simulink model "ElectricalThermalSystemSSC"  (R2026b)
settings: Solver=VariableStepAuto
undefined symbols (not defined in the file): coolant_pipe_D, coolant_valve_D_ratio_max, coolant_valve_D_ratio_min, coolant_valve_displacement, EnvAirTemp, EnvGrvty, PlntThrCabCO2Init, PlntThrCabDucArea, PlntThrCabFanMaxFlw, PlntThrCabHtc, PlntThrCabNPass, PlntThrCabRelHInit, PlntThrCabTempAvg, PlntThrChArea, PlntThrCmpMaxSpd, PlntThrCoolTnkArea, PlntThrCoolTnkVol, PlntThrDoorsArea, PlntThrDoorsK, PlntThrDoorsTk, PlntThrExpDia, PlntThrFanMaxSpd, PlntThrFanMechEff, PlntThrFanVolEff, PlntThrGlassArea, PlntThrGlassK, PlntThrGlassTk, PlntThrHeaterMaxPwr, PlntThrHexNTubes, PlntThrHexTubeDia, PlntThrPipeArea, PlntThrPipeDia, PlntThrPmpMaxSpd, PlntThrPTCLimTemp, PlntThrPTCPwrGain, PlntThrRefrigDia, PlntThrRefrigPinit, PlntThrRoofArea, PlntThrRoofK, PlntThrRoofTk, PlntThrValDisp, PlntThrValDratioMax, PlntThrValDratioMin, PlntThrValRefrDisp, PlntThrValRefrDratio, PlntThrValSplMax, ThrmEM1, ThrmEM2, ThrmEM3, ThrmEM4
libraries: fl_lib x149, nesl_utility x81, SimscapeFluids_lib x35, autolibutils x21
(part 1 of 6)
settings Model: ModifiedByFormat=The MathWorks, Inc.  Creator=The MathWorks, Inc.  LastModifiedBy=The MathWorks, Inc.

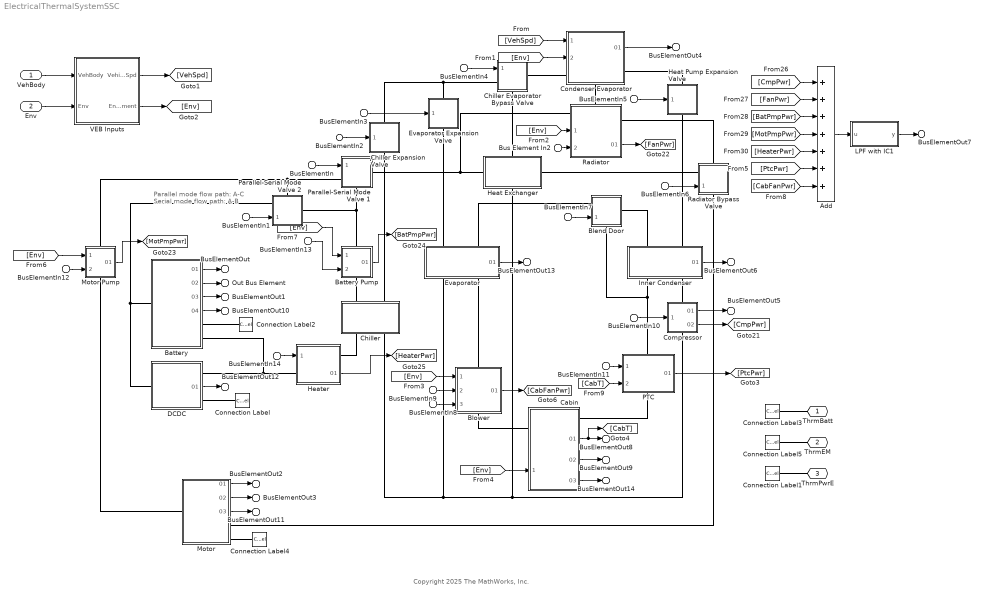
== system ElectricalThermalSystemSSC ==
  note: Parallel mode flow path: A-C
      | Serial mode flow path: A-B
  note: Copyright 2025 The MathWorks, Inc.
  VehBody : Inport
  Env : Inport  Port=2
  BusElementIn10 : Inport  Port=3  PortName=Cntrl  Element=Thermal.CmpCmd
  Bus Element In2 : Inport  Port=3  PortName=Cntrl  Element=Thermal.FanCmd
  BusElementIn14 : Inport  Port=3  PortName=Cntrl  Element=Thermal.HeaterCmd
  BusElementIn12 : Inport  Port=3  PortName=Cntrl  Element=Thermal.MotPmpCmd
  BusElementIn13 : Inport  Port=3  PortName=Cntrl  Element=Thermal.BattPmpCmd
  BusElementIn : Inport  Port=3  PortName=Cntrl  Element=Thermal.SerParCmd
  BusElementIn1 : Inport  Port=3  PortName=Cntrl  Element=Thermal.SerParCmd
  BusElementIn6 : Inport  Port=3  PortName=Cntrl  Element=Thermal.RadByPCmd
  BusElementIn9 : Inport  Port=3  PortName=Cntrl  Element=Thermal.CabFanCmd
  BusElementIn8 : Inport  Port=3  PortName=Cntrl  Element=Thermal.RecircCmd
  BusElementIn11 : Inport  Port=3  PortName=Cntrl  Element=Thermal.PtcCmd
  BusElementIn4 : Inport  Port=3  PortName=Cntrl  Element=Thermal.RfrgByPCmd
  BusElementIn7 : Inport  Port=3  PortName=Cntrl  Element=Thermal.BlndAirCmd
  BusElementIn2 : Inport  Port=3  PortName=Cntrl  Element=Thermal.ChlrXCmd
  BusElementIn3 : Inport  Port=3  PortName=Cntrl  Element=Thermal.AcCmd
  BusElementIn5 : Inport  Port=3  PortName=Cntrl  Element=Thermal.HpXCmd
  Add : Sum  Inputs=+++++++
  Battery : Subsystem  Tag=PublishSubsystem  VariantControl=Mapped
      mask Display: disp(get_param(gcb, 'Name'))
  Battery Pump : Subsystem
      settings: PortSchema="{\"entries\":[{\"content\":{\"sides\":[{\"content\":{\"connectorIds\":[\"In1\",\"In2\"]},\"type\":\"ConnectorPlacement.EquallySpacedRectSide\",\"uuid\":\"8608e54e-2c97-4e6c-91d5-e9fd83f4c634\"},{\"content\":{\"connectorIds\":[\"Out1\"],\"side\":\"RIGHT\"},\"type\":\"ConnectorPlacement.EquallySpacedRectSide\",\"uuid\":\"2094794e-7928-4a36-8d26-6d0877832239\"},{\"content\":{\"connectorIds\":[\"LConn1\"],\"side\":\"TOP\"},\"type\":\"ConnectorPlacement.EquallySpacedRectSide\",\"uuid\":\"5d2e6c3a-6919-4acd-9f23-628827b4d5b1\"},{\"content\":{\"connectorIds\":[\"RConn1\"],\"side\":\"BOTTOM\"},\"type\":\"ConnectorPlacement.EquallySpacedRectSide\",\"uuid\":\"7eb8f1d1-21e2-47d8-bcb5-892664c8f83c\"}]},\"type\":\"ConnectorPlacement.EquallySpacedConnector\",\"uuid\":\"45db803b-5189-4980-a07c-fba0b10a9ca2\"}],\"packageUris\":[\"http://schema.mathworks.com/mf0/Connector/R2020b\"],\"version\":\"1.0\"}"
      mask Display:
      | plot(100*cos(linspace(0, 2*pi, 500)), 100*sin(linspace(0, 2*pi, 500)))
      | patch([0 24 -24 0], [-100 -55 -55 -100]+1, [0 0 0])
  Blend Door : Subsystem
      settings: PortSchema="{\"entries\":[{\"content\":{\"sides\":[{\"content\":{\"connectorIds\":[\"LConn1\",\"In1\"]},\"type\":\"ConnectorPlacement.EquallySpacedRectSide\",\"uuid\":\"8608e54e-2c97-4e6c-91d5-e9fd83f4c634\"},{\"content\":{\"connectorIds\":[\"RConn1\"],\"side\":\"RIGHT\"},\"type\":\"ConnectorPlacement.EquallySpacedRectSide\",\"uuid\":\"2094794e-7928-4a36-8d26-6d0877832239\"},{\"content\":{\"side\":\"TOP\"},\"type\":\"ConnectorPlacement.EquallySpacedRectSide\",\"uuid\":\"5d2e6c3a-6919-4acd-9f23-628827b4d5b1\"},{\"content\":{\"connectorIds\":[\"RConn2\"],\"side\":\"BOTTOM\"},\"type\":\"ConnectorPlacement.EquallySpacedRectSide\",\"uuid\":\"12f1c895-2983-4276-b305-f1b4f2b8f289\"}]},\"type\":\"ConnectorPlacement.EquallySpacedConnector\",\"uuid\":\"45db803b-5189-4980-a07c-fba0b10a9ca2\"}],\"packageUris\":[\"http://schema.mathworks.com/mf0/Connector/R2020b\"],\"version\":\"1.0\"}"
      mask Display:
      | color('white')
      | plot(100, 100)
      | plot(-100, -100)
      | color('black')
      | 
      | plot([0 -100 -100 0], [0 50 -50 0])
      | plot([0 100 100 0], [0 50 -50 0])
      | plot([0 50 -50 0], [0 -100 -100 0])
  Blower : Subsystem  Tag=PublishSubsystem
      settings: PortSchema="{\"entries\":[{\"content\":{\"sides\":[{\"content\":{\"connectorIds\":[\"In1\",\"In2\",\"In3\"]},\"type\":\"ConnectorPlacement.EquallySpacedRectSide\",\"uuid\":\"9f1db8dd-3953-4c85-b0fd-c908a14d75c2\"},{\"content\":{\"connectorIds\":[\"Out1\"],\"side\":\"RIGHT\"},\"type\":\"ConnectorPlacement.EquallySpacedRectSide\",\"uuid\":\"6831d28e-85a7-47d3-a33b-c75afeea3e4b\"},{\"content\":{\"connectorIds\":[\"LConn1\"],\"side\":\"TOP\"},\"type\":\"ConnectorPlacement.EquallySpacedRectSide\",\"uuid\":\"f6a34470-b429-4b8f-bc43-b876cd933588\"},{\"content\":{\"connectorIds\":[\"RConn1\"],\"side\":\"BOTTOM\"},\"type\":\"ConnectorPlacement.EquallySpacedRectSide\",\"uuid\":\"65552e63-bdf8-40c1-9881-c42b86485e87\"}]},\"type\":\"ConnectorPlacement.EquallySpacedConnector\",\"uuid\":\"95b80f6b-f2a0-41c8-b218-6929a9df8903\"}],\"packageUris\":[\"http://schema.mathworks.com/mf0/Connector/R2020b\"],\"version\":\"1.0\"}"
      mask Display:
      | plot(100*cos(linspace(0, 2*pi, 500)), 100*sin(linspace(0, 2*pi, 500)))
      | plot([28 80], [96 -60])
      | plot([-28 -80], [96 -60])
      | patch(-50*sin(3*linspace(0, pi, 500)).*cos(linspace(0, pi, 500)), -50*sin(3*linspace(0, pi, 500)).*sin(linspace(0, pi, 500)), [0 0 0])
  Cabin : Subsystem  Tag=PublishSubsystem
      settings: PortSchema="{\"entries\":[{\"content\":{\"sides\":[{\"content\":{\"connectorIds\":[\"LConn1\",\"In1\"]},\"type\":\"ConnectorPlacement.EquallySpacedRectSide\",\"uuid\":\"20781a4d-44d2-4d8b-9b82-72093275c353\"},{\"content\":{\"connectorIds\":[\"RConn1\",\"Out1\",\"Out2\",\"Out3\"],\"side\":\"RIGHT\"},\"type\":\"ConnectorPlacement.EquallySpacedRectSide\",\"uuid\":\"764c44ca-e93e-4bde-bd39-740c4b6195f1\"},{\"content\":{\"side\":\"TOP\"},\"type\":\"ConnectorPlacement.EquallySpacedRectSide\",\"uuid\":\"542c8f7d-7f76-4cb4-898c-a40529f31b50\"}]},\"type\":\"ConnectorPlacement.EquallySpacedConnector\",\"uuid\":\"d0ad0532-a708-440a-8350-71ab63903cc5\"}],\"packageUris\":[\"http://schema.mathworks.com/mf0/Connector/R2020b\"],\"version\":\"1.0\"}"
      mask Display: disp(get_param(gcb, 'Name'))
  Chiller : Subsystem  Tag=PublishSubsystem
      settings: PortSchema="{\"entries\":[{\"content\":{\"sides\":[{\"content\":{},\"type\":\"ConnectorPlacement.EquallySpacedRectSide\",\"uuid\":\"08dd7f1a-2c57-4e0b-bc0c-3dc595a62f47\"},{\"content\":{\"side\":\"RIGHT\"},\"type\":\"ConnectorPlacement.EquallySpacedRectSide\",\"uuid\":\"ff3adbe6-50e6-4ee9-89c8-33b172e39e14\"},{\"content\":{\"connectorIds\":[\"LConn1\",\"LConn2\"],\"side\":\"TOP\"},\"type\":\"ConnectorPlacement.EquallySpacedRectSide\",\"uuid\":\"dbd0f117-c61e-4d8b-a34c-15c789eeb10d\"},{\"content\":{\"connectorIds\":[\"RConn1\",\"RConn2\"],\"side\":\"BOTTOM\"},\"type\":\"ConnectorPlacement.EquallySpacedRectSide\",\"uuid\":\"0d4c84fc-b13c-4ee0-9956-2ee11d67b2ad\"}]},\"type\":\"ConnectorPlacement.EquallySpacedConnector\",\"uuid\":\"74c2ffb8-8fce-48fb-ac7c-d547444760e2\"}],\"packageUris\":[\"http://schema.mathworks.com/mf0/Connector/R2020b\"],\"version\":\"1.0\"}"
      mask Display: disp(get_param(gcb, 'Name'))
  Chiller Expansion Valve : Subsystem  Tag=PublishSubsystem
      settings: PortSchema="{\"entries\":[{\"content\":{\"sides\":[{\"content\":{\"connectorIds\":[\"In1\"]},\"type\":\"ConnectorPlacement.EquallySpacedRectSide\",\"uuid\":\"8608e54e-2c97-4e6c-91d5-e9fd83f4c634\"},{\"content\":{\"side\":\"RIGHT\"},\"type\":\"ConnectorPlacement.EquallySpacedRectSide\",\"uuid\":\"2094794e-7928-4a36-8d26-6d0877832239\"},{\"content\":{\"connectorIds\":[\"LConn1\"],\"side\":\"TOP\"},\"type\":\"ConnectorPlacement.EquallySpacedRectSide\",\"uuid\":\"5d2e6c3a-6919-4acd-9f23-628827b4d5b1\"},{\"content\":{\"connectorIds\":[\"RConn1\"],\"side\":\"BOTTOM\"},\"type\":\"ConnectorPlacement.EquallySpacedRectSide\",\"uuid\":\"5466525f-0f04-4dbe-888f-4c3dddfbc528\"}]},\"type\":\"ConnectorPlacement.EquallySpacedConnector\",\"uuid\":\"45db803b-5189-4980-a07c-fba0b10a9ca2\"}],\"packageUris\":[\"http://schema.mathworks.com/mf0/Connector/R2020b\"],\"version\":\"1.0\"}"
      mask Display:
      | color('white')
      | plot(100, 100)
      | plot(-100, -100)
      | color('black')
      | 
      | plot([0 50 -50 0], [0 -100 -100 0])
      | plot([0 50 -50 0], [0 100 100 0])
  Chiller Evaporator Bypass Valve : Subsystem  Tag=PublishSubsystem
      settings: PortSchema="{\"entries\":[{\"content\":{\"sides\":[{\"content\":{\"connectorIds\":[\"In1\",\"LConn1\"]},\"type\":\"ConnectorPlacement.EquallySpacedRectSide\",\"uuid\":\"8608e54e-2c97-4e6c-91d5-e9fd83f4c634\"},{\"content\":{\"connectorIds\":[\"RConn1\"],\"side\":\"RIGHT\"},\"type\":\"ConnectorPlacement.EquallySpacedRectSide\",\"uuid\":\"2094794e-7928-4a36-8d26-6d0877832239\"},{\"content\":{\"side\":\"TOP\"},\"type\":\"ConnectorPlacement.EquallySpacedRectSide\",\"uuid\":\"5d2e6c3a-6919-4acd-9f23-628827b4d5b1\"},{\"content\":{\"connectorIds\":[\"RConn2\"],\"side\":\"BOTTOM\"},\"type\":\"ConnectorPlacement.EquallySpacedRectSide\",\"uuid\":\"12f1c895-2983-4276-b305-f1b4f2b8f289\"}]},\"type\":\"ConnectorPlacement.EquallySpacedConnector\",\"uuid\":\"45db803b-5189-4980-a07c-fba0b10a9ca2\"}],\"packageUris\":[\"http://schema.mathworks.com/mf0/Connector/R2020b\"],\"version\":\"1.0\"}"
      mask Display:
      | color('white')
      | plot(100, 100)
      | plot(-100, -100)
      | color('black')
      | 
      | plot([0 -100 -100 0], [0 50 -50 0])
      | plot([0 100 100 0], [0 50 -50 0])
      | plot([0 50 -50 0], [0 -100 -100 0])
  Compressor : Subsystem  Tag=PublishSubsystem
      settings: PortSchema="{\"entries\":[{\"content\":{\"sides\":[{\"content\":{\"connectorIds\":[\"In1\"]},\"type\":\"ConnectorPlacement.EquallySpacedRectSide\",\"uuid\":\"8608e54e-2c97-4e6c-91d5-e9fd83f4c634\"},{\"content\":{\"connectorIds\":[\"Out1\",\"Out2\"],\"side\":\"RIGHT\"},\"type\":\"ConnectorPlacement.EquallySpacedRectSide\",\"uuid\":\"2094794e-7928-4a36-8d26-6d0877832239\"},{\"content\":{\"connectorIds\":[\"LConn1\"],\"side\":\"TOP\"},\"type\":\"ConnectorPlacement.EquallySpacedRectSide\",\"uuid\":\"5d2e6c3a-6919-4acd-9f23-628827b4d5b1\"},{\"content\":{\"connectorIds\":[\"RConn1\"],\"side\":\"BOTTOM\"},\"type\":\"ConnectorPlacement.EquallySpacedRectSide\",\"uuid\":\"ed0a8ac6-4625-4be3-8c8e-84380e16051c\"}]},\"type\":\"ConnectorPlacement.EquallySpacedConnector\",\"uuid\":\"45db803b-5189-4980-a07c-fba0b10a9ca2\"}],\"packageUris\":[\"http://schema.mathworks.com/mf0/Connector/R2020b\"],\"version\":\"1.0\"}"
      mask Display:
      | plot(100*cos(linspace(0, 2*pi, 500)), 100*sin(linspace(0, 2*pi, 500)))
      | plot([28 80], [96 -60])
      | plot([-28 -80], [96 -60])
  Condenser Evaporator : Subsystem  Tag=PublishSubsystem
      settings: PortSchema="{\"entries\":[{\"content\":{\"sides\":[{\"content\":{\"connectorIds\":[\"In1\",\"In2\",\"LConn1\"]},\"type\":\"ConnectorPlacement.EquallySpacedRectSide\",\"uuid\":\"07c3df60-ca73-4a82-8a74-bbe62fbe14d4\"},{\"content\":{\"connectorIds\":[\"Out1\",\"RConn1\"],\"side\":\"RIGHT\"},\"type\":\"ConnectorPlacement.EquallySpacedRectSide\",\"uuid\":\"9db9ae49-9d94-4ce4-9f2f-75754f4c26b5\"},{\"content\":{\"side\":\"TOP\"},\"type\":\"ConnectorPlacement.EquallySpacedRectSide\",\"uuid\":\"fd8c0c23-133d-46ca-bac8-f53d714a10c9\"},{\"content\":{\"connectorIds\":[\"RConn2\"],\"side\":\"BOTTOM\"},\"type\":\"ConnectorPlacement.EquallySpacedRectSide\",\"uuid\":\"1982af02-f04e-4e44-9cd8-4410768eed4d\"}]},\"type\":\"ConnectorPlacement.EquallySpacedConnector\",\"uuid\":\"8e0ae7db-f1f8-46e5-b300-69983ccb91b0\"}],\"packageUris\":[\"http://schema.mathworks.com/mf0/Connector/R2020b\"],\"version\":\"1.0\"}"
      mask Display: disp(get_param(gcb, 'Name'))
  Connection Label : ConnectionLabel  Label=ThrmPwrE
  Connection Label1 : ConnectionLabel  Label=ThrmPwrE
  Connection Label2 : ConnectionLabel  Label=ThrmBatt
  Connection Label3 : ConnectionLabel  Label=ThrmBatt
  Connection Label4 : ConnectionLabel  Label=ThrmEM
  Connection Label5 : ConnectionLabel  Label=ThrmEM
  DCDC : Subsystem
      settings: PortSchema="{\"entries\":[{\"content\":{\"sides\":[{\"content\":{\"connectorIds\":[\"LConn1\"]},\"type\":\"ConnectorPlacement.EquallySpacedRectSide\",\"uuid\":\"39ab4129-79f9-4d3d-8bc5-1c8c0a2ebbde\"},{\"content\":{\"connectorIds\":[\"RConn1\",\"Out1\",\"RConn2\"],\"side\":\"RIGHT\"},\"type\":\"ConnectorPlacement.EquallySpacedRectSide\",\"uuid\":\"b43cfbcd-b0a5-4cd8-a54f-30d93fd1b128\"},{\"content\":{\"side\":\"TOP\"},\"type\":\"ConnectorPlacement.EquallySpacedRectSide\",\"uuid\":\"91742ef5-5184-4832-8e69-68c8acd6160b\"}]},\"type\":\"ConnectorPlacement.EquallySpacedConnector\",\"uuid\":\"413d9595-534c-4f8c-8212-717ae374098d\"}],\"packageUris\":[\"http://schema.mathworks.com/mf0/Connector/R2020b\"],\"version\":\"1.0\"}"
      mask Display: disp(get_param(gcb, 'Name'))
  Evaporator : Subsystem  Tag=PublishSubsystem
      settings: PortSchema="{\"entries\":[{\"content\":{\"sides\":[{\"content\":{},\"type\":\"ConnectorPlacement.EquallySpacedRectSide\",\"uuid\":\"08dd7f1a-2c57-4e0b-bc0c-3dc595a62f47\"},{\"content\":{\"connectorIds\":[\"Out1\"],\"side\":\"RIGHT\"},\"type\":\"ConnectorPlacement.EquallySpacedRectSide\",\"uuid\":\"ff3adbe6-50e6-4ee9-89c8-33b172e39e14\"},{\"content\":{\"connectorIds\":[\"LConn1\",\"LConn2\"],\"side\":\"TOP\"},\"type\":\"ConnectorPlacement.EquallySpacedRectSide\",\"uuid\":\"dbd0f117-c61e-4d8b-a34c-15c789eeb10d\"},{\"content\":{\"connectorIds\":[\"RConn1\",\"RConn2\"],\"side\":\"BOTTOM\"},\"type\":\"ConnectorPlacement.EquallySpacedRectSide\",\"uuid\":\"a1739911-191b-44a6-b898-cc4889767178\"}]},\"type\":\"ConnectorPlacement.EquallySpacedConnector\",\"uuid\":\"74c2ffb8-8fce-48fb-ac7c-d547444760e2\"}],\"packageUris\":[\"http://schema.mathworks.com/mf0/Connector/R2020b\"],\"version\":\"1.0\"}"
      mask Display: disp(get_param(gcb, 'Name'))
  Evaporator Expansion Valve : Subsystem  Tag=PublishSubsystem
      settings: PortSchema="{\"entries\":[{\"content\":{\"sides\":[{\"content\":{\"connectorIds\":[\"In1\"]},\"type\":\"ConnectorPlacement.EquallySpacedRectSide\",\"uuid\":\"8608e54e-2c97-4e6c-91d5-e9fd83f4c634\"},{\"content\":{\"side\":\"RIGHT\"},\"type\":\"ConnectorPlacement.EquallySpacedRectSide\",\"uuid\":\"2094794e-7928-4a36-8d26-6d0877832239\"},{\"content\":{\"connectorIds\":[\"LConn1\"],\"side\":\"TOP\"},\"type\":\"ConnectorPlacement.EquallySpacedRectSide\",\"uuid\":\"5d2e6c3a-6919-4acd-9f23-628827b4d5b1\"},{\"content\":{\"connectorIds\":[\"RConn1\"],\"side\":\"BOTTOM\"},\"type\":\"ConnectorPlacement.EquallySpacedRectSide\",\"uuid\":\"dee56540-0438-4e4d-b3ab-37064a293584\"}]},\"type\":\"ConnectorPlacement.EquallySpacedConnector\",\"uuid\":\"45db803b-5189-4980-a07c-fba0b10a9ca2\"}],\"packageUris\":[\"http://schema.mathworks.com/mf0/Connector/R2020b\"],\"version\":\"1.0\"}"
      mask Display:
      | color('white')
      | plot(100, 100)
      | plot(-100, -100)
      | color('black')
      | 
      | plot([0 50 -50 0], [0 -100 -100 0])
      | plot([0 50 -50 0], [0 100 100 0])
  Heat Exchanger : Subsystem  Tag=PublishSubsystem
      settings: PortSchema="{\"entries\":[{\"content\":{\"sides\":[{\"content\":{\"connectorIds\":[\"LConn1\"]},\"type\":\"ConnectorPlacement.EquallySpacedRectSide\",\"uuid\":\"08dd7f1a-2c57-4e0b-bc0c-3dc595a62f47\"},{\"content\":{\"connectorIds\":[\"RConn1\"],\"side\":\"RIGHT\"},\"type\":\"ConnectorPlacement.EquallySpacedRectSide\",\"uuid\":\"ff3adbe6-50e6-4ee9-89c8-33b172e39e14\"},{\"content\":{\"connectorIds\":[\"LConn2\"],\"side\":\"TOP\"},\"type\":\"ConnectorPlacement.EquallySpacedRectSide\",\"uuid\":\"dbd0f117-c61e-4d8b-a34c-15c789eeb10d\"},{\"content\":{\"connectorIds\":[\"RConn2\"],\"side\":\"BOTTOM\"},\"type\":\"ConnectorPlacement.EquallySpacedRectSide\",\"uuid\":\"042be640-9063-45a3-8f14-0e35b2f9701a\"}]},\"type\":\"ConnectorPlacement.EquallySpacedConnector\",\"uuid\":\"74c2ffb8-8fce-48fb-ac7c-d547444760e2\"}],\"packageUris\":[\"http://schema.mathworks.com/mf0/Connector/R2020b\"],\"version\":\"1.0\"}"
      mask Display: disp(get_param(gcb, 'Name'))
  Heat Pump Expansion Valve : Subsystem  Tag=PublishSubsystem
      settings: PortSchema="{\"entries\":[{\"content\":{\"sides\":[{\"content\":{\"connectorIds\":[\"In1\"]},\"type\":\"ConnectorPlacement.EquallySpacedRectSide\",\"uuid\":\"8608e54e-2c97-4e6c-91d5-e9fd83f4c634\"},{\"content\":{\"side\":\"RIGHT\"},\"type\":\"ConnectorPlacement.EquallySpacedRectSide\",\"uuid\":\"2094794e-7928-4a36-8d26-6d0877832239\"},{\"content\":{\"connectorIds\":[\"LConn1\"],\"side\":\"TOP\"},\"type\":\"ConnectorPlacement.EquallySpacedRectSide\",\"uuid\":\"5d2e6c3a-6919-4acd-9f23-628827b4d5b1\"},{\"content\":{\"connectorIds\":[\"RConn1\"],\"side\":\"BOTTOM\"},\"type\":\"ConnectorPlacement.EquallySpacedRectSide\",\"uuid\":\"a6d8b143-f5c4-47d8-b413-b9e61d8ce1dd\"}]},\"type\":\"ConnectorPlacement.EquallySpacedConnector\",\"uuid\":\"45db803b-5189-4980-a07c-fba0b10a9ca2\"}],\"packageUris\":[\"http://schema.mathworks.com/mf0/Connector/R2020b\"],\"version\":\"1.0\"}"
      mask Display:
      | color('white')
      | plot(100, 100)
      | plot(-100, -100)
      | color('black')
      | 
      | plot([0 50 -50 0], [0 -100 -100 0])
      | plot([0 50 -50 0], [0 100 100 0])
  Heater : Subsystem  Tag=PublishSubsystem
      settings: PortSchema="{\"entries\":[{\"content\":{\"sides\":[{\"content\":{\"connectorIds\":[\"In1\",\"LConn1\"]},\"type\":\"ConnectorPlacement.EquallySpacedRectSide\",\"uuid\":\"cf3791e7-a275-45b9-80b1-f82f6f7fb630\"},{\"content\":{\"connectorIds\":[\"RConn1\",\"Out1\"],\"side\":\"RIGHT\"},\"type\":\"ConnectorPlacement.EquallySpacedRectSide\",\"uuid\":\"ab3b4707-0b89-4b15-a40a-335ce7f1a7d1\"},{\"content\":{\"side\":\"TOP\"},\"type\":\"ConnectorPlacement.EquallySpacedRectSide\",\"uuid\":\"df0da32f-e6fe-4666-9e1f-c9e7ac2aa155\"}]},\"type\":\"ConnectorPlacement.EquallySpacedConnector\",\"uuid\":\"1bf587ca-296b-40b4-a86b-42213e779a2e\"}],\"packageUris\":[\"http://schema.mathworks.com/mf0/Connector/R2020b\"],\"version\":\"1.0\"}"
      mask Display: disp(get_param(gcb, 'Name'))
  Inner Condenser : Subsystem  Tag=PublishSubsystem
      settings: PortSchema="{\"entries\":[{\"content\":{\"sides\":[{\"content\":{},\"type\":\"ConnectorPlacement.EquallySpacedRectSide\",\"uuid\":\"08dd7f1a-2c57-4e0b-bc0c-3dc595a62f47\"},{\"content\":{\"connectorIds\":[\"Out1\"],\"side\":\"RIGHT\"},\"type\":\"ConnectorPlacement.EquallySpacedRectSide\",\"uuid\":\"ff3adbe6-50e6-4ee9-89c8-33b172e39e14\"},{\"content\":{\"connectorIds\":[\"LConn1\",\"LConn2\"],\"side\":\"TOP\"},\"type\":\"ConnectorPlacement.EquallySpacedRectSide\",\"uuid\":\"dbd0f117-c61e-4d8b-a34c-15c789eeb10d\"},{\"content\":{\"connectorIds\":[\"RConn1\",\"RConn2\"],\"side\":\"BOTTOM\"},\"type\":\"ConnectorPlacement.EquallySpacedRectSide\",\"uuid\":\"996ebcad-2560-47a7-9c56-3ae78dd46971\"}]},\"type\":\"ConnectorPlacement.EquallySpacedConnector\",\"uuid\":\"74c2ffb8-8fce-48fb-ac7c-d547444760e2\"}],\"packageUris\":[\"http://schema.mathworks.com/mf0/Connector/R2020b\"],\"version\":\"1.0\"}"
      mask Display: disp(get_param(gcb, 'Name'))
  LPF with IC1 : Subsystem  mask{wc=10, InitCond=0, dataType=off}
      mask prompts: wc "Cutoff frequency, wc [rad/s]"; InitCond "Initial condition, InitCond [same as u]"; dataType "Enforce same input data type"
      mask TypeOptions wc: Cont LPF IC/wc
      mask TypeOptions InitCond: Initial Condition/Value
      mask TypeOptions dataType: Cont LPF IC/dataType
  Motor : Subsystem  Tag=PublishSubsystem
      mask Display: disp(get_param(gcb, 'Name'))
  Motor Pump : Subsystem  Tag=PublishSubsystem
      settings: PortSchema="{\"entries\":[{\"content\":{\"sides\":[{\"content\":{\"connectorIds\":[\"In1\",\"In2\"]},\"type\":\"ConnectorPlacement.EquallySpacedRectSide\",\"uuid\":\"8608e54e-2c97-4e6c-91d5-e9fd83f4c634\"},{\"content\":{\"connectorIds\":[\"Out1\"],\"side\":\"RIGHT\"},\"type\":\"ConnectorPlacement.EquallySpacedRectSide\",\"uuid\":\"2094794e-7928-4a36-8d26-6d0877832239\"},{\"content\":{\"connectorIds\":[\"LConn1\"],\"side\":\"TOP\"},\"type\":\"ConnectorPlacement.EquallySpacedRectSide\",\"uuid\":\"5d2e6c3a-6919-4acd-9f23-628827b4d5b1\"},{\"content\":{\"connectorIds\":[\"RConn1\"],\"side\":\"BOTTOM\"},\"type\":\"ConnectorPlacement.EquallySpacedRectSide\",\"uuid\":\"33b18e2e-1f33-4985-aa8c-29c4f8ccc63e\"}]},\"type\":\"ConnectorPlacement.EquallySpacedConnector\",\"uuid\":\"45db803b-5189-4980-a07c-fba0b10a9ca2\"}],\"packageUris\":[\"http://schema.mathworks.com/mf0/Connector/R2020b\"],\"version\":\"1.0\"}"
      mask Display:
      | plot(100*cos(linspace(0, 2*pi, 500)), 100*sin(linspace(0, 2*pi, 500)))
      | patch([0 24 -24 0], [-100 -55 -55 -100]+1, [0 0 0])
  PTC : Subsystem  Tag=PublishSubsystem
      settings: PortSchema="{\"entries\":[{\"content\":{\"sides\":[{\"content\":{\"connectorIds\":[\"In1\",\"In2\"]},\"type\":\"ConnectorPlacement.EquallySpacedRectSide\",\"uuid\":\"e68f4e4f-d2a0-4f21-a3dd-a8ccea0ce87c\"},{\"content\":{\"connectorIds\":[\"Out1\"],\"side\":\"RIGHT\"},\"type\":\"ConnectorPlacement.EquallySpacedRectSide\",\"uuid\":\"01f15736-e6d7-4b17-9e84-cef8e8356dfe\"},{\"content\":{\"connectorIds\":[\"LConn1\"],\"side\":\"TOP\"},\"type\":\"ConnectorPlacement.EquallySpacedRectSide\",\"uuid\":\"cb1790c7-7993-46e4-a971-f0b801f1d2ca\"},{\"content\":{\"connectorIds\":[\"RConn1\"],\"side\":\"BOTTOM\"},\"type\":\"ConnectorPlacement.EquallySpacedRectSide\",\"uuid\":\"8429c419-0ca8-47a9-96c7-e8d1ee01deb6\"},{\"content\":{\"side\":\"HIDDEN\"},\"type\":\"ConnectorPlacement.EquallySpacedRectSide\",\"uuid\":\"e2e3575c-3b20-453d-a897-62a34bc693b5\"}]},\"type\":\"ConnectorPlacement.EquallySpacedConnector\",\"uuid\":\"0a7b2bb7-4c38-48ec-bfc1-fef0f38ff266\"}],\"packageUris\":[\"http://schema.mathworks.com/mf0/Connector/R2020b\"],\"version\":\"1.0\"}"
      mask Display: disp(get_param(gcb, 'Name'))
  Parallel-Serial Mode Valve 1 : Subsystem  Tag=PublishSubsystem
      settings: PortSchema="{\"entries\":[{\"content\":{\"sides\":[{\"content\":{\"connectorIds\":[\"In1\",\"LConn1\"]},\"type\":\"ConnectorPlacement.EquallySpacedRectSide\",\"uuid\":\"701091b4-901c-43e1-a8a1-50bf4fd327d1\"},{\"content\":{\"connectorIds\":[\"RConn1\"],\"side\":\"RIGHT\"},\"type\":\"ConnectorPlacement.EquallySpacedRectSide\",\"uuid\":\"6ee33cdd-bbd1-4683-8a8c-22edb39550e2\"},{\"content\":{\"side\":\"TOP\"},\"type\":\"ConnectorPlacement.EquallySpacedRectSide\",\"uuid\":\"c0b8be11-b43c-4098-95a0-d44066221ea6\"},{\"content\":{\"connectorIds\":[\"RConn2\"],\"side\":\"BOTTOM\"},\"type\":\"ConnectorPlacement.EquallySpacedRectSide\",\"uuid\":\"08745159-a473-4b1a-b64e-559ffda253bb\"}]},\"type\":\"ConnectorPlacement.EquallySpacedConnector\",\"uuid\":\"9280612b-569a-4615-9ade-e87314c5223e\"}],\"packageUris\":[\"http://schema.mathworks.com/mf0/Connector/R2020b\"],\"version\":\"1.0\"}"
      mask Display:
      | color('white')
      | plot(100, 100)
      | plot(-100, -100)
      | color('black')
      | 
      | plot([0 -100 -100 0], [0 50 -50 0])
      | plot([0 100 100 0], [0 50 -50 0])
      | plot([0 50 -50 0], [0 -100 -100 0])
  Parallel-Serial Mode Valve 2 : Subsystem
      settings: PortSchema="{\"entries\":[{\"content\":{\"sides\":[{\"content\":{\"connectorIds\":[\"LConn1\",\"In1\"]},\"type\":\"ConnectorPlacement.EquallySpacedRectSide\",\"uuid\":\"07c3df60-ca73-4a82-8a74-bbe62fbe14d4\"},{\"content\":{\"connectorIds\":[\"RConn1\"],\"side\":\"RIGHT\"},\"type\":\"ConnectorPlacement.EquallySpacedRectSide\",\"uuid\":\"9db9ae49-9d94-4ce4-9f2f-75754f4c26b5\"},{\"content\":{\"connectorIds\":[\"LConn2\"],\"side\":\"TOP\"},\"type\":\"ConnectorPlacement.EquallySpacedRectSide\",\"uuid\":\"fd8c0c23-133d-46ca-bac8-f53d714a10c9\"}]},\"type\":\"ConnectorPlacement.EquallySpacedConnector\",\"uuid\":\"8e0ae7db-f1f8-46e5-b300-69983ccb91b0\"}],\"packageUris\":[\"http://schema.mathworks.com/mf0/Connector/R2020b\"],\"version\":\"1.0\"}"
      mask Display:
      | color('white')
      | plot(100, 100)
      | plot(-100, -100)
      | color('black')
      | 
      | plot([0 -100 -100 0], [0 50 -50 0])
      | plot([0 100 100 0], [0 50 -50 0])
      | plot([0 50 -50 0], [0 100 100 0])
  Radiator : Subsystem  Tag=PublishSubsystem
      settings: PortSchema="{\"entries\":[{\"content\":{\"sides\":[{\"content\":{\"connectorIds\":[\"LConn1\",\"In1\",\"In2\"]},\"type\":\"ConnectorPlacement.EquallySpacedRectSide\",\"uuid\":\"1c8aa983-a374-4f1b-b303-31d972477bc1\"},{\"content\":{\"connectorIds\":[\"RConn1\",\"Out1\"],\"side\":\"RIGHT\"},\"type\":\"ConnectorPlacement.EquallySpacedRectSide\",\"uuid\":\"9470a7c4-8d01-4f33-b281-130c1633b9af\"},{\"content\":{\"connectorIds\":[\"LConn2\"],\"side\":\"TOP\"},\"type\":\"ConnectorPlacement.EquallySpacedRectSide\",\"uuid\":\"521bcd61-502e-4408-add3-862bd83fd72a\"},{\"content\":{\"side\":\"HIDDEN\"},\"type\":\"ConnectorPlacement.EquallySpacedRectSide\",\"uuid\":\"1fd51896-89cd-4b86-8982-5d9c8888072c\"}]},\"type\":\"ConnectorPlacement.EquallySpacedConnector\",\"uuid\":\"d9db812f-15c4-4875-aa5b-4de8fb002b03\"}],\"packageUris\":[\"http://schema.mathworks.com/mf0/Connector/R2020b\"],\"version\":\"1.0\"}"
      mask Display: disp(get_param(gcb, 'Name'))
  Radiator Bypass Valve : Subsystem  Tag=PublishSubsystem
      settings: PortSchema="{\"entries\":[{\"content\":{\"sides\":[{\"content\":{\"connectorIds\":[\"LConn1\",\"In1\"]},\"type\":\"ConnectorPlacement.EquallySpacedRectSide\",\"uuid\":\"701091b4-901c-43e1-a8a1-50bf4fd327d1\"},{\"content\":{\"side\":\"RIGHT\"},\"type\":\"ConnectorPlacement.EquallySpacedRectSide\",\"uuid\":\"6ee33cdd-bbd1-4683-8a8c-22edb39550e2\"},{\"content\":{\"connectorIds\":[\"LConn2\"],\"side\":\"TOP\"},\"type\":\"ConnectorPlacement.EquallySpacedRectSide\",\"uuid\":\"c0b8be11-b43c-4098-95a0-d44066221ea6\"},{\"content\":{\"connectorIds\":[\"RConn1\"],\"side\":\"BOTTOM\"},\"type\":\"ConnectorPlacement.EquallySpacedRectSide\",\"uuid\":\"83027471-d1d2-4b40-ac40-09f8b2d5e483\"}]},\"type\":\"ConnectorPlacement.EquallySpacedConnector\",\"uuid\":\"9280612b-569a-4615-9ade-e87314c5223e\"}],\"packageUris\":[\"http://schema.mathworks.com/mf0/Connector/R2020b\"],\"version\":\"1.0\"}"
      mask Display:
      | color('white')
      | plot(100, 100)
      | plot(-100, -100)
      | color('black')
      | 
      | plot([0 -100 -100 0], [0 50 -50 0])
      | plot([0 50 -50 0], [0 100 100 0])
      | plot([0 50 -50 0], [0 -100 -100 0])
  VEB Inputs : Subsystem
  ThrmBatt : PMIOPort  Side=Left
  ThrmEM : PMIOPort  Port=2  Side=Left
  ThrmPwrE : PMIOPort  Port=3  Side=Left
  BusElementOut3 : Outport  PortName=Thermal  Element=EMCoolTempOut
  BusElementOut : Outport  PortName=Thermal  Element=BattTemp
  BusElementOut2 : Outport  PortName=Thermal  Element=MotorTemp
  BusElementOut4 : Outport  PortName=Thermal  Element=CondPress
  BusElementOut7 : Outport  PortName=Thermal  Element=EAccPwr
  Out Bus Element : Outport  PortName=Thermal  Element=BattCoolTemp
  BusElementOut10 : Outport  PortName=Thermal  Element=Qbatt
  BusElementOut12 : Outport  PortName=Thermal  Element=Qpwre
  BusElementOut11 : Outport  PortName=Thermal  Element=Qem
  BusElementOut1 : Outport  PortName=Thermal  Element=BattCoolMFlw
  BusElementOut5 : Outport  PortName=Thermal  Element=EvapPress
  BusElementOut8 : Outport  PortName=Thermal  Element=CabTemp
  BusElementOut6 : Outport  PortName=Thermal  Element=CabCondPr
  BusElementOut9 : Outport  PortName=Thermal  Element=CabVntTemp
  BusElementOut14 : Outport  PortName=Thermal  Element=CabRelH
  BusElementOut13 : Outport  PortName=Thermal  Element=EvapVntTemp
  wires:
  Battery/4(04) -> BusElementOut10/1
  Battery/3(03) -> BusElementOut1/1
  Battery/2(02) -> Out Bus Element/1
  Battery/1(01) -> BusElementOut/1
  Motor/1(01) -> BusElementOut2/1
  Motor/2(02) -> BusElementOut3/1
  Env/1 -> VEB Inputs/2(Env)
  VehBody/1 -> VEB Inputs/1(VehBody)
  VEB Inputs/2(Environment) -> [Env]
  VEB Inputs/1(VehicleSpd) -> [VehSpd]
  [VehSpd] -> Condenser Evaporator/1(1)
  [Env] -> Condenser Evaporator/2(2)
  Condenser Evaporator/1(01) -> BusElementOut4/1
  [Env] -> Radiator/1(1)
  Bus Element In2/1 -> Radiator/2(2)
  BusElementIn/1 -> Parallel-Serial Mode Valve 1/1(1)
  BusElementIn1/1 -> Parallel-Serial Mode Valve 2/1(1)
  BusElementIn2/1 -> Chiller Expansion Valve/1(1)
  BusElementIn3/1 -> Evaporator Expansion Valve/1(1)
  BusElementIn4/1 -> Chiller Evaporator Bypass Valve/1(1)
  BusElementIn5/1 -> Heat Pump Expansion Valve/1(1)
  BusElementIn6/1 -> Radiator Bypass Valve/1(1)
  BusElementIn7/1 -> Blend Door/1(1)
  Compressor/1(01) -> BusElementOut5/1
  Inner Condenser/1(01) -> BusElementOut6/1
  [Env] -> Blower/1(1)
  BusElementIn8/1 -> Blower/3(3)
  BusElementIn9/1 -> Blower/2(2)
  LPF with IC1/1(y) -> BusElementOut7/1
  Add/1 -> LPF with IC1/1(u)
  [CabFanPwr] -> Add/7
  Blower/1(01) -> [CabFanPwr]
  Cabin/1(01) -> [CabT], BusElementOut8/1
  Cabin/2(02) -> BusElementOut9/1
  [Env] -> Cabin/1(1)
  BusElementIn10/1 -> Compressor/1(1)
  Compressor/2(02) -> [CmpPwr]
  [CmpPwr] -> Add/1
  Radiator/1(01) -> [FanPwr]
  [FanPwr] -> Add/2
  Motor/3(03) -> BusElementOut11/1
  DCDC/1(01) -> BusElementOut12/1
  PTC/1(01) -> [PtcPwr]
  BusElementIn11/1 -> PTC/1(1)
  [PtcPwr] -> Add/6
  [Env] -> Motor Pump/1(1)
  [Env] -> Battery Pump/1(1)
  BusElementIn12/1 -> Motor Pump/2(2)
  BusElementIn13/1 -> Battery Pump/2(2)
  BusElementIn14/1 -> Heater/1(1)
  Cabin/3(03) -> BusElementOut14/1
  [BatPmpPwr] -> Add/3
  [MotPmpPwr] -> Add/4
  [HeaterPwr] -> Add/5
  Battery Pump/1(01) -> [BatPmpPwr]
  Motor Pump/1(01) -> [MotPmpPwr]
  Heater/1(01) -> [HeaterPwr]
  [CabT] -> PTC/2(2)
  Evaporator/1(01) -> BusElementOut13/1
  connections:
  Battery/RConn2 -- DCDC/RConn1 -- Heater/LConn1
  Parallel-Serial Mode Valve 2/LConn1 -- Battery/LConn1 -- DCDC/LConn1
  Parallel-Serial Mode Valve 2/LConn2 -- Motor Pump/LConn1 -- Parallel-Serial Mode Valve 1/LConn1
  Chiller Expansion Valve/LConn1 -- Chiller Evaporator Bypass Valve/LConn1 -- Evaporator Expansion Valve/LConn1
  Battery Pump/LConn1 -- Parallel-Serial Mode Valve 2/RConn1 -- Parallel-Serial Mode Valve 1/RConn2
  Heat Exchanger/LConn1 -- Parallel-Serial Mode Valve 1/RConn1 -- Radiator/LConn1
  Inner Condenser/RConn1 -- PTC/LConn1 -- Blend Door/RConn2
  Heat Exchanger/RConn2 -- Evaporator/RConn1 -- Chiller/RConn2 -- Compressor/RConn1
  Battery/RConn1 -- Connection Label2/LConn1
  Radiator Bypass Valve/RConn1 -- Motor/RConn1
  Blend Door/RConn1 -- Inner Condenser/LConn1
  Battery Pump/RConn1 -- Chiller/LConn1
  Evaporator/LConn1 -- Evaporator Expansion Valve/RConn1
  Radiator/LConn2 -- Condenser Evaporator/RConn2
  Inner Condenser/LConn2 -- Heat Pump Expansion Valve/RConn1
  Radiator Bypass Valve/LConn2 -- Radiator/RConn1
  Chiller/RConn1 -- Heater/RConn1
  Radiator Bypass Valve/LConn1 -- Heat Exchanger/RConn1
  Condenser Evaporator/RConn1 -- Heat Pump Expansion Valve/LConn1
  Blend Door/LConn1 -- Evaporator/LConn2
  Chiller Evaporator Bypass Valve/RConn1 -- Condenser Evaporator/LConn1
  Blower/RConn1 -- Cabin/LConn1
  Chiller Evaporator Bypass Valve/RConn2 -- Heat Exchanger/LConn2
  Chiller/LConn2 -- Chiller Expansion Valve/RConn1
  Blower/LConn1 -- Evaporator/RConn2
  Inner Condenser/RConn2 -- Compressor/LConn1
  Motor Pump/RConn1 -- Motor/LConn1
  ThrmBatt/RConn1 -- Connection Label3/LConn1
  ThrmEM/RConn1 -- Connection Label5/LConn1
  Connection Label4/LConn1 -- Motor/RConn2
  ThrmPwrE/RConn1 -- Connection Label1/LConn1
  Connection Label/LConn1 -- DCDC/RConn2
  PTC/RConn1 -- Cabin/RConn1

== system ElectricalThermalSystemSSC/Battery ==
  Batt Cool1 : fl_lib/Thermal/Thermal Elements/Thermal Mass  mass_type=foundation.enum.constant_variable.constant  mass=10 kg  sp_heat=PlntThrBattPlateCp J/(K*kg)  mass_min=1e-6 kg  num_ports=foundation.enum.numPorts2.two  m_specify=off  m_priority=High  m=1 kg  m_nominal_specify=off  m_nominal_value=1  m_nominal_unit=kg  T_specify=on  T_priority=High  T=EnvAirTemp K  T_nominal_specify=off  T_nominal_value=1  T_nominal_unit=K  Q_specify=off  Q_priority=None  Q=0 W  Q_nominal_specify=off  Q_nominal_value=1  Q_nominal_unit=W
  Coolant Jacket 1 : SimscapeFluids_lib/Thermal Liquid/Pipes & Fittings/Pipe (TL)  dynamic_compressibility=simscape.enum.onoff.on  inertia=simscape.enum.onoff.off  num_segments=1  pipe_length=PlntThrBattJacLen m  cross_section_geometry=fluids.thermal_liquid.pipes_fittings.enum.CrossSectionGeometry.Custom  pipe_diameter=0.1 m  pipe_inner_diameter=0.05 m  pipe_outer_diameter=0.1 m  pipe_width=0.1 m  pipe_height=0.1 m  pipe_major_axis=0.1 m  pipe_minor_axis=0.05 m  pipe_side=0.1 m  pipe_angle=30 deg  area=4*PlntThrChArea m^2  Dh=PlntThrChDia m  annular_heat_transfer_walls=fluids.thermal_liquid.pipes_fittings.enum.AnnularPipeWalls.AnnularInner  elevation_spec=foundation.enum.constant_variable.constant  elevation_gain=0 m  gravity_spec=foundation.enum.constant_variable.constant  g=EnvGrvty m/s^2  pressure_loss_spec=fluids.thermal_liquid.pipes_fittings.enum.PressureLossSpec.Haaland  local_pressure_loss_spec=fluids.thermal_liquid.pipes_fittings.enum.LocalLossSpec.AggregateLength  length_add=0 m  loss_coefficient=0.1  roughness_spec=fluids.thermal_liquid.pipes_fittings.enum.RoughnessSpec.Custom  roughness=1.5e-5 m  Re_friction_TLU=[ 400 1000 1.5e+3 3e+3 4e+3 6e+3 1e+4 2e+4 4e+4 6e+4 1e+5 1e+8 ]  friction_factor_TLU=[ 0.264 0.112 0.07099999999999999 0.0417 0.0387 0.0268 0.025 0.0232 0.0226 0.022 0.0214 0.0214 ]  Re_lam=100  Re_tur=500  shape_factor=64  mdot_nominal=[ 0.1 1 ] kg/s  p_diff_nominal=[ 0.001 0.01 ] MPa  mdot_threshold=1e-6 kg/s  wall_spec=fluids.thermal_liquid.pipes_fittings.enum.wall_spec.rigid  vol_expansion_spec=fluids.thermal_liquid.pipes_fittings.enum.VolumeExpansionSpec.Diameter  area_pressure_gain=1e-6 m^2/MPa  static_pressure_TLU=[.1, 1] MPa  area_pressure_gain_TLU=[1e-05, 1.1e-05] m^2  material_behavior_spec=fluids.thermal_liquid.pipes_fittings.enum.PipeMaterialBehavior.Linear  diameter_pressure_gain=1.2e-6 m/MPa  wall_thickness=0.05 m  elastic_modulus=69 GPa  stress_TLU=[276, 310] MPa  strain_TLU=[.004, .02]  stress_assert_action=simscape.enum.assert.action.none  stress_max=400 MPa  poisson_ratio=0.33  wall_time_constant=0.01 s  environment_spec=foundation.enum.pressure_spec.atmospheric  environment_pressure=0.101325 MPa  thermal_expansion=false  alpha_L_wall=24 um/(deltaK*m)  thermal_expansion_Tref=293.15 K  heat_transfer_spec=fluids.thermal_liquid.pipes_fittings.enum.HeatTransferSpec.DittusBoelter  mdot_nominal_heat=[ 0.1 1 ] kg/s  T_in_nominal=[ 293.15 293.15 ] K  T_out_nominal=[ 300 300 ] K  p_in_nominal_heat=[ 0.101325 0.101325 ] MPa  T_wall_nominal=[ 303.15 303.15 ] K  T_wall_eff_nominal=[303.15, 303.15] K  a_coeff=0.3  b_Re_power=0.8  c_Pr_power=0.33  Nu_lam=3.66  Re_Colburn_TLU=[ 100 150 1000 ]  Colburn_factor_TLU=[ 0.019 0.013 0.002 ]  Re_Nu_TLU=[ 100 150 1000 ]  Pr_Nu_TLU=[ 1 10 ]  Nu_TLU=[ 3.72 4.21; 3.75 4.44; 4.21 7.15 ]  annular_correction=fluids.thermal_liquid.pipes_fittings.enum.AnnularPipeCorrectionFactor.Gnielinski  p0_vec=EnvAbsPrs Pa  T0_vec=EnvAirTemp K  mdot0=0.1 kg/s  p_nominal=0.101325 MPa  T_nominal=293.15 K
  Flow Resistance (TL) : fl_lib/Thermal Liquid/Elements/Flow Resistance (TL)  delta_p_nominal=50 Pa  mdot_nominal=0.02 kg/s  area=PlntThrPipeArea m^2  laminar_fraction=1e-3
  Flow Resistance (TL)1 : fl_lib/Thermal Liquid/Elements/Flow Resistance (TL)  delta_p_nominal=50 Pa  mdot_nominal=0.02 kg/s  area=PlntThrPipeArea m^2  laminar_fraction=1e-3
  S1 : Subsystem
      settings: PortSchema="{\"entries\":[{\"content\":{\"sides\":[{\"content\":{\"connectorIds\":[\"LConn1\"]},\"type\":\"ConnectorPlacement.EquallySpacedRectSide\",\"uuid\":\"61532473-bcb1-48d4-ba77-0f0975f199f2\"},{\"content\":{\"connectorIds\":[\"Out1\",\"RConn1\",\"Out2\"],\"side\":\"RIGHT\"},\"type\":\"ConnectorPlacement.EquallySpacedRectSide\",\"uuid\":\"dbd252db-2a33-4b3b-9cdd-a592642b7899\"},{\"content\":{\"side\":\"TOP\"},\"type\":\"ConnectorPlacement.EquallySpacedRectSide\",\"uuid\":\"da4820fc-3b0e-48e2-98b2-5d19cd2de8cb\"}]},\"type\":\"ConnectorPlacement.EquallySpacedConnector\",\"uuid\":\"adcbdcfb-b681-4304-a7c1-16e7936a1963\"}],\"packageUris\":[\"http://schema.mathworks.com/mf0/Connector/R2020b\"],\"version\":\"1.0\"}"
      mask Display: disp(get_param(gcb, 'Name'))
  SC1 : Subsystem
      mask Display: disp(get_param(gcb, 'Name'))
  Simscape Bus2 : SimscapeBus  HierarchyStrings=ThrmBatt1
  B : PMIOPort  Side=Left
  T : PMIOPort  Port=2  Side=Right
  A : PMIOPort  Port=3  Side=Right
  01 : Outport
  02 : Outport  Port=2
  03 : Outport  Port=3
  04 : Outport  Port=4
  wires:
  S1/2(H) -> 04/1
  SC1/2(BattCoolMFlw) -> 03/1
  SC1/1(BattCoolTemp) -> 02/1
  S1/1(BattTemp) -> 01/1
  connections:
  Batt Cool1/LConn1 -- S1/RConn1
  Flow Resistance (TL)1/RConn1 -- SC1/RConn1
  A/RConn1 -- Flow Resistance (TL)1/LConn1
  Batt Cool1/RConn1 -- Simscape Bus2/LConn1
  S1/LConn1 -- Coolant Jacket 1/LConn2
  SC1/LConn1 -- Coolant Jacket 1/LConn1
  Flow Resistance (TL)/RConn1 -- B/RConn1
  Coolant Jacket 1/RConn1 -- Flow Resistance (TL)/LConn1
  T/RConn1 -- Simscape Bus2/RConn1

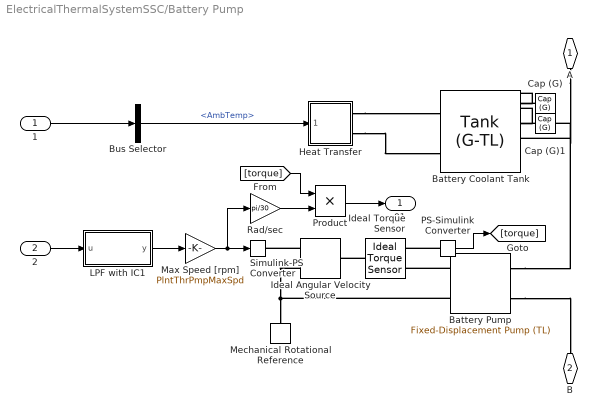
== system ElectricalThermalSystemSSC/Battery Pump ==
  1 : Inport
  2 : Inport  Port=2
  Battery Coolant Tank : SimscapeFluids_lib/Thermal Liquid/Tanks & Accumulators/Tank (G-TL)  num_inlet=2  volume_total=PlntThrCoolTnkVol l  volume_spec=1  tank_area=PlntThrCoolTnkArea m^2  level_TLU=[0, 3, 5] m  volume_TLU=[0, 4, 6] m^3  inlet_areas_A1B1=[.01, .01] m^2  inlet_height_A2=0.1 m  inlet_area_A2=0.01 m^2  inlet_heights_A2B2=[0, 0] m  inlet_areas_A2B2=[1 1] * PlntThrPipeArea m^2  inlet_heights_A2B2C2=[.1, .05, 0] m  inlet_areas_A2B2C2=[.01, .01, .01] m^2  inlet_heights_A2B2C2D2=0.1 * ones(1, 4) m  inlet_areas_A2B2C2D2=0.01 * ones(1, 4) m^2  inlet_heights_A2B2C2D2E2=0.1 * ones(1, 5) m  inlet_areas_A2B2C2D2E2=0.01 * ones(1, 5) m^2  inlet_heights_A2B2C2D2E2F2=0.1 * ones(1, 6) m  inlet_areas_A2B2C2D2E2F2=0.01 * ones(1, 6) m^2  capacity_check=0  max_liquid_capacity=coolant_tank_volume l  g=0 m/s^2  level_specify=on  level_priority=None  level=5 m  level_nominal_specify=off  level_nominal_value=1  level_nominal_unit=m  volume_liquid_specify=on  volume_liquid_priority=High  volume_liquid=0.5 * PlntThrCoolTnkVol l  volume_liquid_nominal_specify=off  volume_liquid_nominal_value=1  volume_liquid_nominal_unit=m^3  mass_liquid_specify=off  mass_liquid_priority=None  mass_liquid=5e+3 kg  mass_liquid_nominal_specify=off  mass_liquid_nominal_value=1  mass_liquid_nominal_unit=kg  T_liquid_specify=on  T_liquid_priority=High  T_liquid=EnvAirTemp K  T_liquid_nominal_specify=off  T_liquid_nominal_value=1  T_liquid_nominal_unit=K  p_gas_specify=on  p_gas_priority=High  p_gas=EnvAbsPrs Pa  p_gas_nominal_specify=off  p_gas_nominal_value=1  p_gas_nominal_unit=MPa  T_gas_specify=on  T_gas_priority=High  T_gas=EnvAirTemp K  T_gas_nominal_specify=off  T_gas_nominal_value=1  T_gas_nominal_unit=K  rho_gas_specify=off  rho_gas_priority=None  rho_gas=1.2 kg/m^3  rho_gas_nominal_specify=off  rho_gas_nominal_value=1  rho_gas_nominal_unit=kg/m^3
  Battery Pump : SimscapeFluids_lib/Thermal Liquid/Pumps & Motors/Fixed-Displacement Pump (TL)  loss_spec=1  displacement=PlntThrPmpDisp l/rev  omega_nominal=0.5 * PlntThrPmpMaxSpd rpm  p_nominal=0.1 MPa  mu_nominal=0.9 cP  vol_eff_nominal=0.92  mech_eff_nominal=0.88  no_load_torque=0.03 N*m  p_diff_eff_TLU=[.1, 1, 2] MPa  omega_eff_TLU=[25, 50, 100, 200, 300, 400] rad/s  vol_eff_TLU=[.816, .908, .954, .977, .981, .984; .325, .663, .831, .916, .925, .946; .137, .568, .78, .892, .893, .91]  mech_eff_TLU=[.996, .996, .996, .996, .996, .996; .988, .989, .989, .989, .989, .99; .981, .981, .982, .982, .983, .984]  p_diff_loss_TLU=[.1, 1, 2] MPa  omega_loss_TLU=[25, 50, 100, 200, 300, 400] rad/s  vol_loss_TLU=[.023, .023, .023, .023, .0285, .032; .0844, .0842, .0845, .084, .1125, .108; .1079, .108, .11, .108, .1605, .18] * 1e-3 m^3/s  mech_loss_TLU=[.002, .002, .002, .002, .002, .002; .0607, .0556, .0556, .0556, .0556, .0505; .1937, .1937, .1833, .1833, .1729, .1626] N*m  vol_eff_min=1e-3  vol_eff_max=1  mech_eff_min=1e-3  mech_eff_max=1  pressure_threshold=1e-3 MPa  omega_threshold=10 rad/s  area=PlntThrPipeArea m^2  supplied_range_check=0  pump_mode_check=simscape.enum.assert.action.none  pressure_check=simscape.enum.assert.action.none  p_min_valid=0.101325 MPa
  Bus Selector : BusSelector  OutputSignals=AmbTemp
  Cap (G) : fl_lib/Gas/Elements/Cap (G)  p_specify=off  p_priority=None  p=0.101325 MPa  p_nominal_specify=off  p_nominal_value=1  p_nominal_unit=MPa  T_specify=off  T_priority=None  T=293.15 K  T_nominal_specify=off  T_nominal_value=1  T_nominal_unit=K
  Cap (G)1 : fl_lib/Gas/Elements/Cap (G)  p_specify=off  p_priority=None  p=0.101325 MPa  p_nominal_specify=off  p_nominal_value=1  p_nominal_unit=MPa  T_specify=off  T_priority=None  T=293.15 K  T_nominal_specify=off  T_nominal_value=1  T_nominal_unit=K
  Heat Transfer : Subsystem
  Ideal Angular Velocity Source : fl_lib/Mechanical/Mechanical Sources/Ideal Angular Velocity Source
  Ideal Torque Sensor : fl_lib/Mechanical/Mechanical Sensors/Ideal Torque Sensor
  LPF with IC1 : Subsystem  mask{wc=1, InitCond=0, dataType=off}
      mask prompts: wc "Cutoff frequency, wc [rad/s]"; InitCond "Initial condition, InitCond [same as u]"; dataType "Enforce same input data type"
      mask TypeOptions wc: Cont LPF IC/wc
      mask TypeOptions InitCond: Initial Condition/Value
      mask TypeOptions dataType: Cont LPF IC/dataType
  Max Speed [rpm] : Gain  Gain=PlntThrPmpMaxSpd
  Mechanical Rotational Reference : fl_lib/Mechanical/Rotational Elements/Mechanical Rotational Reference
  PS-Simulink Converter : nesl_utility/PS-Simulink Converter  PhysicalDomain=network_engine_domain  SubClassName=ps_output  LeftPortType=input  RightPortType=output  PseudoPeriodic=off  Frequencies=[]  VectorFormat=inherit  Unit=N*m  AffineConversion=off
  Product : Product
  Rad/sec : Gain  Gain=pi/30
  Simulink-PS Converter : nesl_utility/Simulink-PS Converter  PhysicalDomain=network_engine_domain  SubClassName=ps_input  LeftPortType=input  RightPortType=output  PseudoPeriodic=off  Frequencies=[]  NoiseDistribution=none  NoiseParameters=[]  Unit=rpm  AffineConversion=off  FilteringAndDerivatives=provide  SimscapeFilterOrder=1  InputFilterTimeConstant=0.001  UdotUserProvided=0
  A : PMIOPort  Side=Left
  B : PMIOPort  Port=2  Side=Right
  01 : Outport
  wires:
  2/1 -> LPF with IC1/1(u)
  Bus Selector/1 -> Heat Transfer/1(1)  "<AmbTemp>"
  1/1 -> Bus Selector/1
  LPF with IC1/1(y) -> Max Speed [rpm]/1
  Max Speed [rpm]/1 -> Rad/sec/1, Simulink-PS Converter/1
  PS-Simulink Converter/1 -> [torque]
  Rad/sec/1 -> Product/2
  [torque] -> Product/1
  Product/1 -> 01/1
  connections:
  Ideal Angular Velocity Source/RConn2 -- Battery Pump/RConn2 -- Mechanical Rotational Reference/LConn1
  Battery Pump/LConn2 -- B/RConn1
  A/RConn1 -- Battery Coolant Tank/LConn3
  Cap (G)1/LConn1 -- Battery Coolant Tank/LConn2
  Heat Transfer/RConn2 -- Battery Coolant Tank/RConn2
  Cap (G)/LConn1 -- Battery Coolant Tank/LConn1
  Battery Pump/LConn1 -- Battery Coolant Tank/LConn4
  Heat Transfer/RConn1 -- Battery Coolant Tank/RConn1
  Ideal Angular Velocity Source/RConn1 -- Simulink-PS Converter/RConn1
  Ideal Torque Sensor/LConn1 -- Ideal Angular Velocity Source/LConn1
  Battery Pump/RConn1 -- Ideal Torque Sensor/RConn1
  PS-Simulink Converter/LConn1 -- Ideal Torque Sensor/RConn2

== system ElectricalThermalSystemSSC/Blend Door ==
  1 : Inport
  Blend Door : Subsystem  Tag=PublishSubsystem  mask{min_area=1e-8 * PlntThrCabDucArea, max_area=0.9 * PlntThrCabDucArea, port_area=PlntThrCabDucArea, Cd=0.8, tau=1}
      mask prompts: min_area "Min restriction area (m^2)"; max_area "Max restriction area (m^2)"; port_area "Cross-sectional area at ports A, B, and C (m^2)"; Cd "Discharge coefficient"; tau "Opening time constant (s)"
      settings: PortSchema="{\"entries\":[{\"content\":{\"sides\":[{\"content\":{\"connectorIds\":[\"LConn1\",\"In1\"]},\"type\":\"ConnectorPlacement.EquallySpacedRectSide\",\"uuid\":\"701091b4-901c-43e1-a8a1-50bf4fd327d1\"},{\"content\":{\"connectorIds\":[\"RConn1\"],\"side\":\"RIGHT\"},\"type\":\"ConnectorPlacement.EquallySpacedRectSide\",\"uuid\":\"6ee33cdd-bbd1-4683-8a8c-22edb39550e2\"},{\"content\":{\"side\":\"TOP\"},\"type\":\"ConnectorPlacement.EquallySpacedRectSide\",\"uuid\":\"c0b8be11-b43c-4098-95a0-d44066221ea6\"},{\"content\":{\"connectorIds\":[\"RConn2\"],\"side\":\"BOTTOM\"},\"type\":\"ConnectorPlacement.EquallySpacedRectSide\",\"uuid\":\"1c585638-1e64-4636-940b-c407bc21f999\"}]},\"type\":\"ConnectorPlacement.EquallySpacedConnector\",\"uuid\":\"9280612b-569a-4615-9ade-e87314c5223e\"}],\"packageUris\":[\"http://schema.mathworks.com/mf0/Connector/R2020b\"],\"version\":\"1.0\"}"
  A : PMIOPort  Side=Left
  B : PMIOPort  Port=2  Side=Right
  C : PMIOPort  Port=3  Side=Right
  wires:
  1/1 -> Blend Door/1(cmd)
  connections:
  Blend Door/LConn1 -- A/RConn1
  B/RConn1 -- Blend Door/RConn1
  C/RConn1 -- Blend Door/RConn2
